simulink model "PID_based_control_model"  (R2015a)
settings: Solver=ode45  StartTime=0.0  StopTime=300  RelTol=1e-3
libraries: simulink x1, powerlib x1
settings Model: Creator=HP  LastModifiedBy=HP

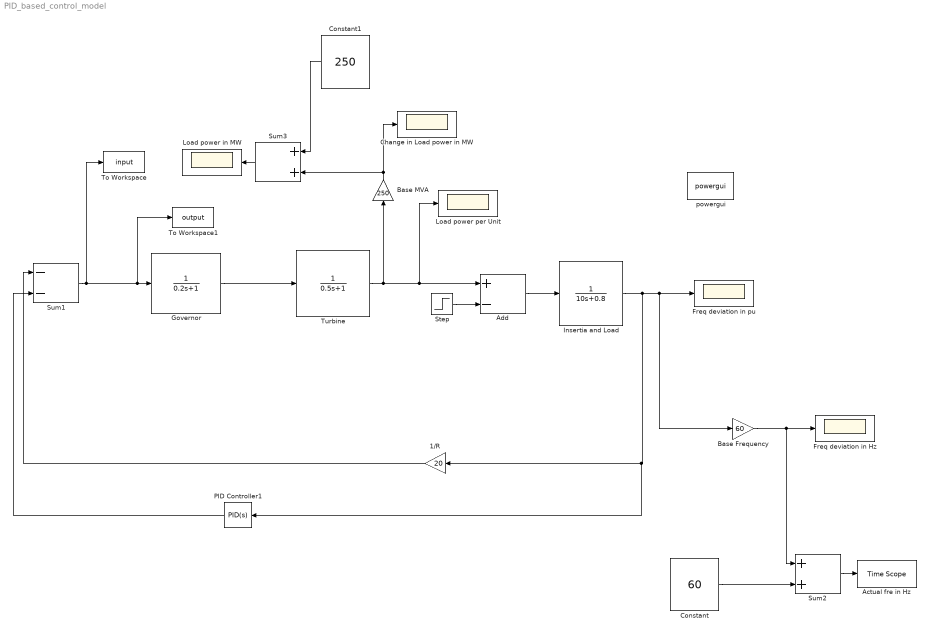
== system PID_based_control_model ==
  1/R : Gain  Gain=20
  Actual fre in Hz : TimeScope
  Add : Sum  Inputs=+-
  Base Frequency : Gain  Gain=60
  Base MVA : Gain  Gain=250
  Change in Load power in MW : Scope
      settings: SaveName=ScopeData4
  Constant : Constant  Value=60
  Constant1 : Constant  Value=250
  Freq deviation in Hz : Scope
  Freq deviation in pu : Scope
  Governor : TransferFcn  Denominator=[0.2 1]
  Insertia and Load : TransferFcn  Denominator=[10 0.8]
  Load power in MW : Scope
      settings: YMin=299  YMax=301  SaveName=ScopeData5
  Load power per Unit : Scope
      settings: SaveName=ScopeData3
  PID Controller1 : simulink/Continuous/PID Controller  Controller=PID  TimeDomain=Continuous-time  SampleTime=-1  IntegratorMethod=Forward Euler  FilterMethod=Forward Euler  Form=Parallel  UseFilter=on  ControllerParametersSource=internal  P=50  I=30  D=10  N=100  InitialConditionSource=internal  InitialConditionForIntegrator=0  InitialConditionForFilter=0  ExternalReset=none  LimitOutput=off  UpperSaturationLimit=inf  LowerSaturationLimit=-inf  LinearizeAsGain=on  AntiWindupMode=none  Kb=1  TrackingMode=off  Kt=1  PParamMin=[]  PParamMax=[]  IParamMin=[]  IParamMax=[]  DParamMin=[]  DParamMax=[]  NParamMin=[]  NParamMax=[]  KbParamMin=[]  KbParamMax=[]  KtParamMin=[]  KtParamMax=[]  POutMin=[]  POutMax=[]  IOutMin=[]  IOutMax=[]  DOutMin=[]  DOutMax=[]  NOutMin=[]  NOutMax=[]  KbOutMin=[]  KbOutMax=[]  KtOutMin=[]  KtOutMax=[]  IntegratorOutMin=[]  IntegratorOutMax=[]  FilterOutMin=[]  FilterOutMax=[]  SumOutMin=[]  SumOutMax=[]  SumI1OutMin=[]  SumI1OutMax=[]  SumI2OutMin=[]  SumI2OutMax=[]  SumI3OutMin=[]  SumI3OutMax=[]  SumDOutMin=[]  SumDOutMax=[]  SaturationOutMin=[]  SaturationOutMax=[]  IntegratorContinuousStateAttributes=''  IntegratorStateMustResolveToSignalObject=off  IntegratorRTWStateStorageClass=Auto  FilterContinuousStateAttributes=''  FilterStateMustResolveToSignalObject=off  FilterRTWStateStorageClass=Auto  DifferentiatorICPrevScaledInput=0  DifferentiatorOutMin=[]  DifferentiatorOutMax=[]
  Step : Step  Time=100  Before=0.2  After=0.2  SampleTime=0
  Sum1 : Sum  Inputs=--
  Sum2 : Sum
  Sum3 : Sum
  To Workspace : ToWorkspace  VariableName=input  SampleTime=-1
  To Workspace1 : ToWorkspace  VariableName=output  SampleTime=-1
  Turbine : TransferFcn  Denominator=[0.5 1]
  powergui : powerlib/powergui  Priority=1  SimulationMode=Continuous  SolverType=Tustin/Backward Euler (TBE)  SampleTime=50e-6  frequency=60  SPID=off  DisableSnubberDevices=off  DisableRonSwitches=off  DisableVfSwitches=off  SwTol=0  DisplayEquations=off  Interpol=off  methode=off  Ts=100  FunctionMessages=off  echomessages=off  HookPort=off  EnableUseOfTLC=off  x0status=blocks  frequencyindice=60  Pbase=100e6  ErrMax=1e-4  Iterations=50  UnitsV=kV  UnitsW=MW  buscounter=0  RestoreLinks=warning  ResistiveCurrentMeasurement=off  Frange=[0:2:500]  Ylog=off  Xlog=on  ShowGrid=off  save=off  variable=ZData  structure=0  ZoomFFT=off  StartTime=0.0  cycles=1  DisplayStyle=1  fundamental=60  FreqAxis=off  MaxFrequency=1000  frequencyindicesteady=1  RmsSteady=1  display=off
  wires:
  Governor/1 -> Turbine/1
  Add/1 -> Insertia and Load/1
  Step/1 -> Add/2
  Turbine/1 -> Load power per Unit/1, Add/1, Base MVA/1
  Base Frequency/1 -> Sum2/1, Freq deviation in Hz/1
  Constant/1 -> Sum2/2
  Sum2/1 -> Actual fre in Hz/1
  Base MVA/1 -> Change in Load power in MW/1, Sum3/2
  Constant1/1 -> Sum3/1
  Sum3/1 -> Load power in MW/1
  1/R/1 -> Sum1/1
  Sum1/1 -> To Workspace1/1, Governor/1, To Workspace/1
  Insertia and Load/1 -> PID Controller1/1, 1/R/1, Base Frequency/1, Freq deviation in pu/1
  PID Controller1/1 -> Sum1/2
